simulink model "inductionmotor"  (Simulink 7.1)
settings: Solver=ode23tb  StartTime=0.0  StopTime=50  MaxStep=1e-3  RelTol=1e-3
settings Model: Creator=218  LastModifiedBy=jagan
settings OptimizationCC: InitFltsAndDblsToZero=off

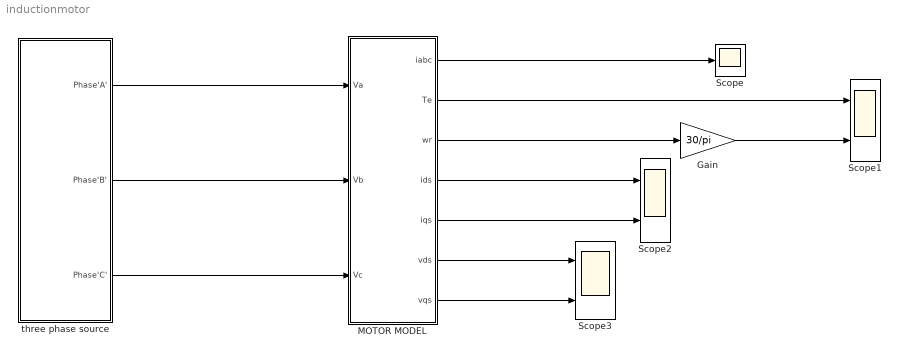
== system inductionmotor ==
  Gain : Gain  Gain=30/pi  ParameterDataType=fixdt(1, 16)  ParameterScaling=2^0  OutDataType=fixdt(1, 16)  OutScaling=2^0
  MOTOR MODEL : Subsystem
  Scope : Scope
  Scope1 : Scope  NumInputPorts=2
      settings: TimeRange=100  YMin=-600~-250  YMax=800~0  SaveName=ScopeData2
  Scope2 : Scope  NumInputPorts=2
      settings: YMin=-5~-5  YMax=5~5  SaveName=ScopeData3
  Scope3 : Scope  NumInputPorts=2
      settings: YMin=-5~-5  YMax=5~5  SaveName=ScopeData4
  three phase source : Subsystem
  wires:
  MOTOR MODEL/2(Te) -> Scope1/1
  MOTOR MODEL/4(ids) -> Scope2/1
  MOTOR MODEL/5(iqs) -> Scope2/2
  MOTOR MODEL/6(vds) -> Scope3/1
  MOTOR MODEL/7(vqs) -> Scope3/2
  Gain/1 -> Scope1/2
  MOTOR MODEL/3(wr) -> Gain/1
  three phase source/1(Phase'A') -> MOTOR MODEL/1(Va)
  three phase source/2(Phase'B') -> MOTOR MODEL/2(Vb)
  three phase source/3(Phase'C') -> MOTOR MODEL/3(Vc)
  MOTOR MODEL/1(iabc) -> Scope/1

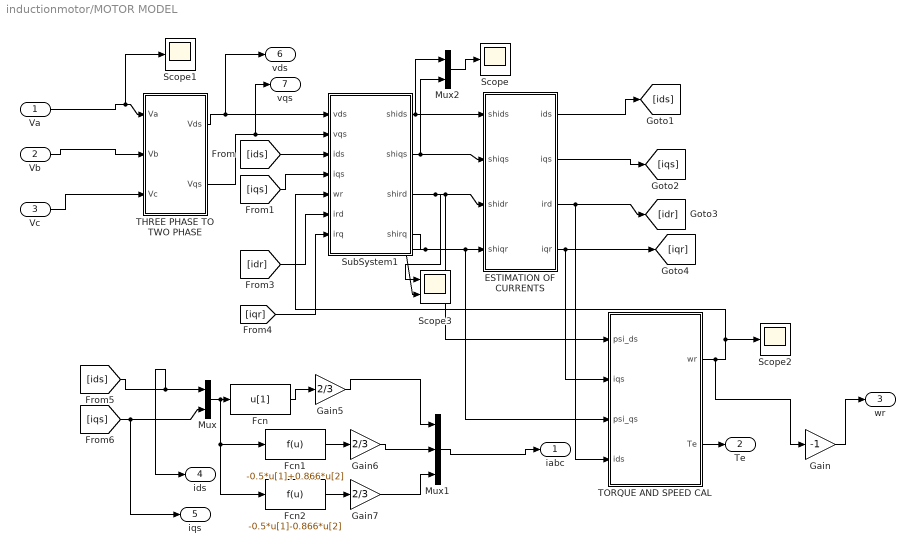
== system inductionmotor/MOTOR MODEL ==
  Va : Inport  OutDataType=sfix(16)  OutScaling=2^0
  Vb : Inport  Port=2  OutDataType=sfix(16)  OutScaling=2^0
  Vc : Inport  Port=3  OutDataType=sfix(16)  OutScaling=2^0
  ESTIMATION OF CURRENTS : Subsystem  mask{Lm=60.6639e-3, Lr=63.456e-3, Ls=62.6956e-3}
  Fcn : Fcn  Expr=u[1]
  Fcn1 : Fcn  Expr=-0.5*u[1]+0.866*u[2]
  Fcn2 : Fcn  Expr=-0.5*u[1]-0.866*u[2]
  Gain : Gain  Gain=-1  ParameterDataType=fixdt(1, 16)  ParameterScaling=2^0  OutDataType=fixdt(1, 16)  OutScaling=2^0
  Gain5 : Gain  Gain=2/3  ParameterDataType=sfix(16)  ParameterScaling=2^0  OutDataType=sfix(16)  OutScaling=2^0  SaturateOnIntegerOverflow=on  OutDataTypeStr=Inherit: Same as input  ParamDataTypeStr=Inherit: Same as input
  Gain6 : Gain  Gain=2/3  ParameterDataType=sfix(16)  ParameterScaling=2^0  OutDataType=sfix(16)  OutScaling=2^0  SaturateOnIntegerOverflow=on  OutDataTypeStr=Inherit: Same as input  ParamDataTypeStr=Inherit: Same as input
  Gain7 : Gain  Gain=2/3  ParameterDataType=sfix(16)  ParameterScaling=2^0  OutDataType=sfix(16)  OutScaling=2^0  SaturateOnIntegerOverflow=on  OutDataTypeStr=Inherit: Same as input  ParamDataTypeStr=Inherit: Same as input
  Mux : Mux  Inputs=2
  Mux1 : Mux  Inputs=3
  Mux2 : Mux  Inputs=2
  Scope : Scope
      settings: TimeRange=0.5  YMin=-1.05  YMax=-0.05
  Scope1 : Scope
      settings: YMin=-450  YMax=450
  Scope2 : Scope
      settings: TimeRange=2  YMin=83  YMax=103
  Scope3 : Scope  NumInputPorts=2
      settings: TimeRange=0.5  YMin=-1.05~-5  YMax=-0.05~5  SaveName=ScopeData7
  SubSystem1 : Subsystem  mask{Rr=0.2447, Rs=0.1589}
  THREE PHASE TO TWO PHASE : Subsystem
  TORQUE AND SPEED CAL : Subsystem  mask{J=2.018}
  iabc : Outport  OutDataType=sfix(16)  OutScaling=2^0
  Te : Outport  Port=2  OutDataType=sfix(16)  OutScaling=2^0
  wr : Outport  Port=3  OutDataType=sfix(16)  OutScaling=2^0
  ids : Outport  Port=4  OutDataType=sfix(16)  OutScaling=2^0
  iqs : Outport  Port=5  OutDataType=sfix(16)  OutScaling=2^0
  vds : Outport  Port=6  OutDataType=sfix(16)  OutScaling=2^0
  vqs : Outport  Port=7  OutDataType=sfix(16)  OutScaling=2^0
  wires:
  THREE PHASE TO TWO PHASE/1(Vds) -> SubSystem1/1(vds), vds/1
  THREE PHASE TO TWO PHASE/2(Vqs) -> SubSystem1/2(vqs), vqs/1
  SubSystem1/3(shird) -> ESTIMATION OF CURRENTS/3(shidr), TORQUE AND SPEED CAL/1(psi_ds), Scope3/1
  SubSystem1/4(shirq) -> ESTIMATION OF CURRENTS/4(shiqr), TORQUE AND SPEED CAL/3(psi_qs), Scope3/2
  [idr] -> SubSystem1/6(ird)
  [iqr] -> SubSystem1/7(irq)
  ESTIMATION OF CURRENTS/3(ird) -> [idr], TORQUE AND SPEED CAL/4(ids)
  ESTIMATION OF CURRENTS/2(iqs) -> [iqs]
  ESTIMATION OF CURRENTS/1(ids) -> [ids]
  [iqs] -> SubSystem1/4(iqs)
  [ids] -> SubSystem1/3(ids)
  SubSystem1/1(shids) -> Mux2/1, ESTIMATION OF CURRENTS/1(shids)
  SubSystem1/2(shiqs) -> Mux2/2, ESTIMATION OF CURRENTS/2("shiqs ")
  Mux2/1 -> Scope/1
  Va/1 -> THREE PHASE TO TWO PHASE/1(Va), Scope1/1
  Vb/1 -> THREE PHASE TO TWO PHASE/2(Vb)
  Vc/1 -> THREE PHASE TO TWO PHASE/3(Vc)
  [ids] -> Mux/1, ids/1
  [iqs] -> Mux/2, iqs/1
  Fcn1/1 -> Gain6/1
  Fcn2/1 -> Gain7/1
  Mux/1 -> Fcn/1, Fcn1/1, Fcn2/1
  Fcn/1 -> Gain5/1
  Gain7/1 -> Mux1/3
  ESTIMATION OF CURRENTS/4(iqr) -> [iqr], TORQUE AND SPEED CAL/2(iqs)
  TORQUE AND SPEED CAL/2(Te) -> Te/1
  Mux1/1 -> iabc/1
  Gain5/1 -> Mux1/1
  Gain6/1 -> Mux1/2
  TORQUE AND SPEED CAL/1(wr) -> Scope2/1, SubSystem1/5(wr), Gain/1
  Gain/1 -> wr/1

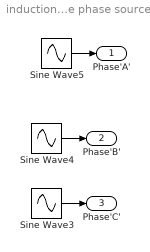
== system inductionmotor/three phase source ==
  Sine Wave3 : Sin  Amplitude=380  Frequency=100*pi  Phase=-2*pi/3
  Sine Wave4 : Sin  Amplitude=380  Frequency=100*pi  Phase=2*pi/3
  Sine Wave5 : Sin  Amplitude=380  Frequency=100*pi
  Phase'A' : Outport
  Phase'B' : Outport  Port=2
  Phase'C' : Outport  Port=3
  wires:
  Sine Wave5/1 -> Phase'A'/1
  Sine Wave4/1 -> Phase'B'/1
  Sine Wave3/1 -> Phase'C'/1

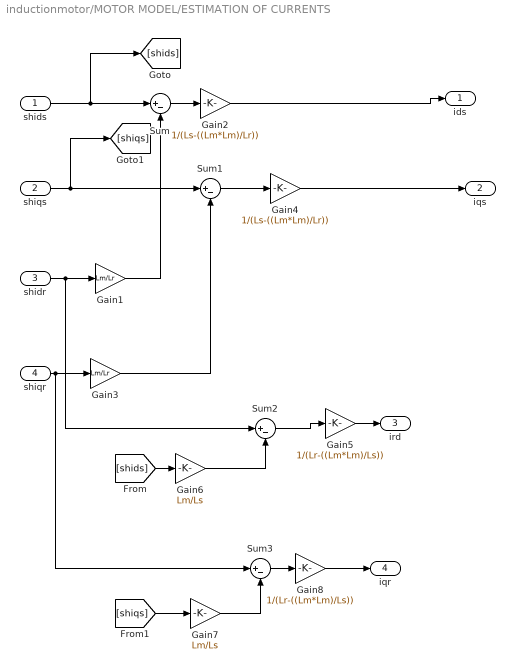
== system inductionmotor/MOTOR MODEL/ESTIMATION OF CURRENTS ==
  shids : Inport  OutDataType=sfix(16)  OutScaling=2^0
  "shiqs " : Inport  Port=2  OutDataType=sfix(16)  OutScaling=2^0
  shidr : Inport  Port=3  OutDataType=sfix(16)  OutScaling=2^0
  shiqr : Inport  Port=4  OutDataType=sfix(16)  OutScaling=2^0
  Gain1 : Gain  Gain=Lm/Lr  ParameterDataType=sfix(16)  ParameterScaling=2^0  OutDataType=sfix(16)  OutScaling=2^0  SaturateOnIntegerOverflow=on  OutDataTypeStr=Inherit: Same as input  ParamDataTypeStr=Inherit: Same as input
  Gain2 : Gain  Gain=1/(Ls-((Lm*Lm)/Lr))  ParameterDataType=sfix(16)  ParameterScaling=2^0  OutDataType=sfix(16)  OutScaling=2^0  SaturateOnIntegerOverflow=on  OutDataTypeStr=Inherit: Same as input  ParamDataTypeStr=Inherit: Same as input
  Gain3 : Gain  Gain=Lm/Lr  ParameterDataType=sfix(16)  ParameterScaling=2^0  OutDataType=sfix(16)  OutScaling=2^0  SaturateOnIntegerOverflow=on  OutDataTypeStr=Inherit: Same as input  ParamDataTypeStr=Inherit: Same as input
  Gain4 : Gain  Gain=1/(Ls-((Lm*Lm)/Lr))  ParameterDataType=sfix(16)  ParameterScaling=2^0  OutDataType=sfix(16)  OutScaling=2^0  SaturateOnIntegerOverflow=on  OutDataTypeStr=Inherit: Same as input  ParamDataTypeStr=Inherit: Same as input
  Gain5 : Gain  Gain=1/(Lr-((Lm*Lm)/Ls))  ParameterDataType=sfix(16)  ParameterScaling=2^0  OutDataType=sfix(16)  OutScaling=2^0  SaturateOnIntegerOverflow=on  OutDataTypeStr=Inherit: Same as input  ParamDataTypeStr=Inherit: Same as input
  Gain6 : Gain  Gain=Lm/Ls  ParameterDataType=sfix(16)  ParameterScaling=2^0  OutDataType=sfix(16)  OutScaling=2^0  SaturateOnIntegerOverflow=on  OutDataTypeStr=Inherit: Same as input  ParamDataTypeStr=Inherit: Same as input
  Gain7 : Gain  Gain=Lm/Ls  ParameterDataType=sfix(16)  ParameterScaling=2^0  OutDataType=sfix(16)  OutScaling=2^0  SaturateOnIntegerOverflow=on  OutDataTypeStr=Inherit: Same as input  ParamDataTypeStr=Inherit: Same as input
  Gain8 : Gain  Gain=1/(Lr-((Lm*Lm)/Ls))  ParameterDataType=sfix(16)  ParameterScaling=2^0  OutDataType=sfix(16)  OutScaling=2^0  SaturateOnIntegerOverflow=on  OutDataTypeStr=Inherit: Same as input  ParamDataTypeStr=Inherit: Same as input
  Sum{,1..3} (4 alike) : Sum  Inputs=|+-  OutDataType=sfix(16)  OutScaling=2^0  SaturateOnIntegerOverflow=on  InputSameDT=on  OutDataTypeStr=Inherit: Same as first input
  ids : Outport  OutDataType=sfix(16)  OutScaling=2^0
  iqs : Outport  Port=2  OutDataType=sfix(16)  OutScaling=2^0
  ird : Outport  Port=3  OutDataType=sfix(16)  OutScaling=2^0
  iqr : Outport  Port=4  OutDataType=sfix(16)  OutScaling=2^0
  wires:
  Gain1/1 -> Sum/2
  Sum/1 -> Gain2/1
  Gain2/1 -> ids/1
  Sum1/1 -> Gain4/1
  Gain3/1 -> Sum1/2
  Gain4/1 -> iqs/1
  Sum2/1 -> Gain5/1
  Gain5/1 -> ird/1
  Gain6/1 -> Sum2/2
  shidr/1 -> Gain1/1, Sum2/1
  Gain7/1 -> Sum3/2
  shiqr/1 -> Gain3/1, Sum3/1
  Sum3/1 -> Gain8/1
  Gain8/1 -> iqr/1
  shids/1 -> Sum/1, [shids]
  [shids] -> Gain6/1
  "shiqs "/1 -> [shiqs], Sum1/1
  [shiqs] -> Gain7/1

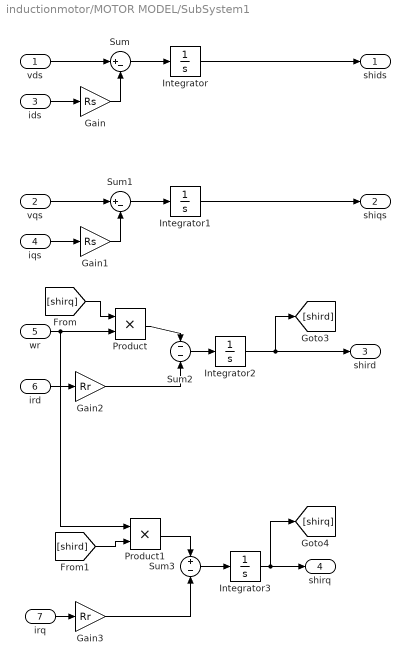
== system inductionmotor/MOTOR MODEL/SubSystem1 ==
  vds : Inport  OutDataType=sfix(16)  OutScaling=2^0
  vqs : Inport  Port=2  OutDataType=sfix(16)  OutScaling=2^0
  ids : Inport  Port=3  OutDataType=sfix(16)  OutScaling=2^0
  iqs : Inport  Port=4  OutDataType=sfix(16)  OutScaling=2^0
  wr : Inport  Port=5  OutDataType=sfix(16)  OutScaling=2^0
  ird : Inport  Port=6  OutDataType=sfix(16)  OutScaling=2^0
  irq : Inport  Port=7  OutDataType=sfix(16)  OutScaling=2^0
  Gain : Gain  Gain=Rs  ParameterDataType=sfix(16)  ParameterScaling=2^0  OutDataType=sfix(16)  OutScaling=2^0  SaturateOnIntegerOverflow=on  OutDataTypeStr=Inherit: Same as input  ParamDataTypeStr=Inherit: Same as input
  Gain1 : Gain  Gain=Rs  ParameterDataType=sfix(16)  ParameterScaling=2^0  OutDataType=sfix(16)  OutScaling=2^0  SaturateOnIntegerOverflow=on  OutDataTypeStr=Inherit: Same as input  ParamDataTypeStr=Inherit: Same as input
  Gain2 : Gain  Gain=Rr  ParameterDataType=sfix(16)  ParameterScaling=2^0  OutDataType=sfix(16)  OutScaling=2^0  SaturateOnIntegerOverflow=on  OutDataTypeStr=Inherit: Same as input  ParamDataTypeStr=Inherit: Same as input
  Gain3 : Gain  Gain=Rr  ParameterDataType=sfix(16)  ParameterScaling=2^0  OutDataType=sfix(16)  OutScaling=2^0  SaturateOnIntegerOverflow=on  OutDataTypeStr=Inherit: Same as input  ParamDataTypeStr=Inherit: Same as input
  Integrator{,1..3} (4 alike) : Integrator
  Product : Product  OutDataType=sfix(16)  OutScaling=2^0  SaturateOnIntegerOverflow=on  InputSameDT=on  OutDataTypeStr=Inherit: Same as first input
  Product1 : Product  OutDataType=sfix(16)  OutScaling=2^0  SaturateOnIntegerOverflow=on  InputSameDT=on  OutDataTypeStr=Inherit: Same as first input
  Sum : Sum  Inputs=|+-  OutDataType=sfix(16)  OutScaling=2^0  SaturateOnIntegerOverflow=on  InputSameDT=on  OutDataTypeStr=Inherit: Same as first input
  Sum1 : Sum  Inputs=|+-  OutDataType=sfix(16)  OutScaling=2^0  SaturateOnIntegerOverflow=on  InputSameDT=on  OutDataTypeStr=Inherit: Same as first input
  Sum2 : Sum  Inputs=--  OutDataType=sfix(16)  OutScaling=2^0  SaturateOnIntegerOverflow=on  InputSameDT=on  OutDataTypeStr=Inherit: Same as first input
  Sum3 : Sum  Inputs=+-  OutDataType=sfix(16)  OutScaling=2^0  SaturateOnIntegerOverflow=on  InputSameDT=on  OutDataTypeStr=Inherit: Same as first input
  shids : Outport  OutDataType=sfix(16)  OutScaling=2^0
  shiqs : Outport  Port=2  OutDataType=sfix(16)  OutScaling=2^0
  shird : Outport  Port=3  OutDataType=sfix(16)  OutScaling=2^0
  shirq : Outport  Port=4  OutDataType=sfix(16)  OutScaling=2^0
  wires:
  vds/1 -> Sum/1
  Gain/1 -> Sum/2
  Sum/1 -> Integrator/1
  vqs/1 -> Sum1/1
  Gain1/1 -> Sum1/2
  Sum1/1 -> Integrator1/1
  ids/1 -> Gain/1
  iqs/1 -> Gain1/1
  ird/1 -> Gain2/1
  Product/1 -> Sum2/1
  Gain2/1 -> Sum2/2
  Sum2/1 -> Integrator2/1
  [shirq] -> Product/1
  wr/1 -> Product/2, Product1/1
  [shird] -> Product1/2
  Product1/1 -> Sum3/1
  irq/1 -> Gain3/1
  Gain3/1 -> Sum3/2
  Sum3/1 -> Integrator3/1
  Integrator2/1 -> shird/1, [shird]
  Integrator1/1 -> shiqs/1
  Integrator/1 -> shids/1
  Integrator3/1 -> shirq/1, [shirq]

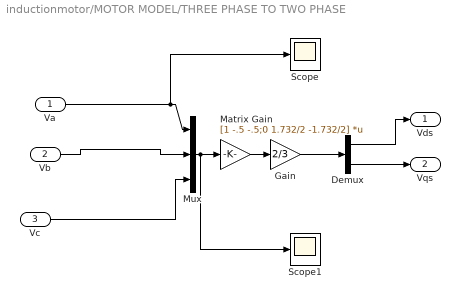
== system inductionmotor/MOTOR MODEL/THREE PHASE TO TWO PHASE ==
  Va : Inport  OutDataType=sfix(16)  OutScaling=2^0
  Vb : Inport  Port=2  OutDataType=sfix(16)  OutScaling=2^0
  Vc : Inport  Port=3  OutDataType=sfix(16)  OutScaling=2^0
  Demux : Demux  Outputs=2
  Gain : Gain  Gain=2/3  ParameterDataType=sfix(16)  ParameterScaling=2^0  OutDataType=sfix(16)  OutScaling=2^0  SaturateOnIntegerOverflow=on  OutDataTypeStr=Inherit: Same as input  ParamDataTypeStr=Inherit: Same as input
  Matrix Gain : Gain  Gain=[1 -.5 -.5;0 1.732/2 -1.732/2]  Multiplication=Matrix(K*u)  ParameterDataType=sfix(16)  ParameterScaling=2^0  OutDataType=sfix(16)  OutScaling=2^0  SaturateOnIntegerOverflow=on  OutDataTypeStr=Inherit: Same as input  ParamDataTypeStr=Inherit: Same as input
  Mux : Mux  Inputs=3
  Scope : Scope
      settings: YMin=-250  YMax=250
  Scope1 : Scope
      settings: TimeRange=0.04  YMin=-250  YMax=250  SaveName=ScopeData5
  Vds : Outport  OutDataType=sfix(16)  OutScaling=2^0
  Vqs : Outport  Port=2  OutDataType=sfix(16)  OutScaling=2^0
  wires:
  Matrix Gain/1 -> Gain/1
  Demux/2 -> Vqs/1
  Demux/1 -> Vds/1
  Mux/1 -> Scope1/1, Matrix Gain/1
  Va/1 -> Mux/1, Scope/1
  Vb/1 -> Mux/2
  Vc/1 -> Mux/3
  Gain/1 -> Demux/1

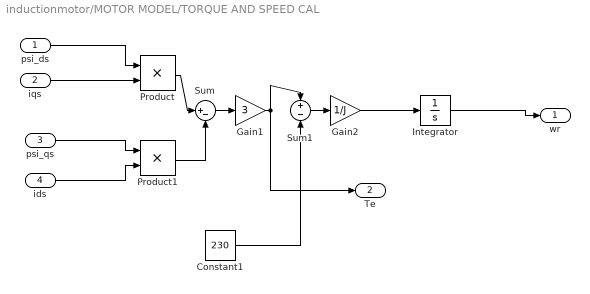
== system inductionmotor/MOTOR MODEL/TORQUE AND SPEED CAL ==
  psi_ds : Inport  OutDataType=sfix(16)  OutScaling=2^0
  iqs : Inport  Port=2  OutDataType=sfix(16)  OutScaling=2^0
  psi_qs : Inport  Port=3  OutDataType=sfix(16)  OutScaling=2^0
  ids : Inport  Port=4  OutDataType=sfix(16)  OutScaling=2^0
  Constant1 : Constant  Value=230  OutDataType=fixdt(1, 16)  OutScaling=2^0
  Gain1 : Gain  Gain=3  ParameterDataType=sfix(16)  ParameterScaling=2^0  OutDataType=sfix(16)  OutScaling=2^0  SaturateOnIntegerOverflow=on  OutDataTypeStr=Inherit: Same as input  ParamDataTypeStr=Inherit: Same as input
  Gain2 : Gain  Gain=1/J  ParameterDataType=sfix(16)  ParameterScaling=2^0  OutDataType=sfix(16)  OutScaling=2^0  SaturateOnIntegerOverflow=on  OutDataTypeStr=Inherit: Same as input  ParamDataTypeStr=Inherit: Same as input
  Integrator : Integrator
  Product : Product  OutDataType=sfix(16)  OutScaling=2^0  SaturateOnIntegerOverflow=on  InputSameDT=on  OutDataTypeStr=Inherit: Same as first input
  Product1 : Product  OutDataType=sfix(16)  OutScaling=2^0  SaturateOnIntegerOverflow=on  InputSameDT=on  OutDataTypeStr=Inherit: Same as first input
  Sum : Sum  Inputs=|+-  OutDataType=sfix(16)  OutScaling=2^0  SaturateOnIntegerOverflow=on  InputSameDT=on  OutDataTypeStr=Inherit: Same as first input
  Sum1 : Sum  Inputs=+-  OutDataType=sfix(16)  OutScaling=2^0  SaturateOnIntegerOverflow=on  InputSameDT=on  OutDataTypeStr=Inherit: Same as first input
  wr : Outport  OutDataType=sfix(16)  OutScaling=2^0
  Te : Outport  Port=2  OutDataType=sfix(16)  OutScaling=2^0
  wires:
  Product/1 -> Sum/1
  Product1/1 -> Sum/2
  Sum/1 -> Gain1/1
  psi_ds/1 -> Product/1
  iqs/1 -> Product/2
  psi_qs/1 -> Product1/1
  ids/1 -> Product1/2
  Gain1/1 -> Te/1, Sum1/1
  Sum1/1 -> Gain2/1
  Gain2/1 -> Integrator/1
  Integrator/1 -> wr/1
  Constant1/1 -> Sum1/2
